simulink model "kopter_se_zavazim_LQR"  (R2024b)
settings: Solver=ode4  StartTime=0.0  StopTime=16  FixedStep=Ts  RelTol=1e-3
values from neighbouring files (symbols this model uses):
  Ac = double(Ac)    [odvozeni_stavova_regulace_a_LQR.m]
  b_moment = 3.6e-7    (= 3.6e-07)    [parametry_kopter_se_zavazim.m]
  Bc = double(Bc)    [odvozeni_stavova_regulace_a_LQR.m]
  Cc = eye(8, 16)    [odvozeni_stavova_regulace_a_LQR.m]
  d = 1    [parametry_kopter_se_zavazim.m]
  Dc = 0    [odvozeni_stavova_regulace_a_LQR.m]
  init_int_dref_lqr = -Ki_lqr\((Uinit-Us)+Kp_lqr*(Xinit_ss-Xs))    [odvozeni_stavova_regulace_a_LQR.m]
  init_int_ref_lqr = -Ki_lqr\(Kp_lqr*xss+uss)    [odvozeni_stavova_regulace_a_LQR.m]
  Ip = m*d^2    (= 1)    [parametry_kopter_se_zavazim.m]
  Ixx = 0.0222    [parametry_kopter_se_zavazim.m]
  Iyy = 0.0222    [parametry_kopter_se_zavazim.m]
  Izz = 0.0429    [parametry_kopter_se_zavazim.m]
  k_thrust = 9.3e-6    (= 9.3e-06)    [parametry_kopter_se_zavazim.m]
  Ki_lqr = K_ex_lqr(:, 17:20)    [odvozeni_stavova_regulace_a_LQR.m]
  Kp_lqr = K_ex_lqr(:, 1:16)    [odvozeni_stavova_regulace_a_LQR.m]
  l = 0.2051    [parametry_kopter_se_zavazim.m]
  M = 2    [parametry_kopter_se_zavazim.m]
  m = 1    [parametry_kopter_se_zavazim.m]
  R_kalman = diag([repmat(1e-2, 1, 3), repmat(7e-4, 1, 3), repmat(3e-4, 1, 2)])    [odvozeni_stavova_regulace_a_LQR.m]
  Ts = 0.01    [odvozeni_stavova_regulace_a_LQR.m]
  Us = [(M+m)*g; 0; 0; 0]    [parametry_kopter_se_zavazim.m]
  Xinit_ss = [Xinit_matrix; [0 0 0 0 0 0 0 0]']    [parametry_kopter_se_zavazim.m]
  Xs = [0;0;0; 0;0;0; 0;0; 0;0;0; 0;0;0; 0;0]    [parametry_kopter_se_zavazim.m]
undefined symbols (not defined in the file or in its folder): Continuous, L, Time
libraries: simulink_extras x11, ctrlSharedLib x2, simulink x2
(part 1 of 3)
settings Model: Creator=Admin  LastModifiedBy=Admin

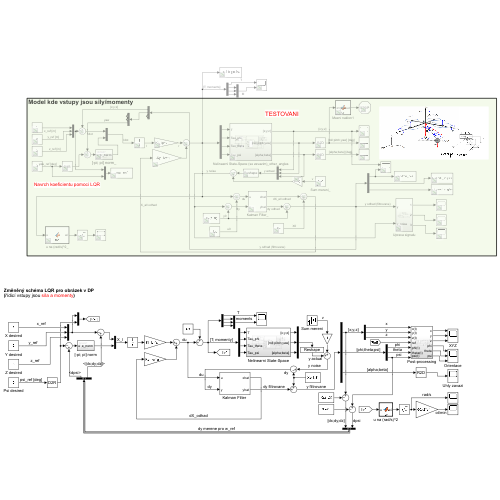
[thumbnail: Simulink's stored preview of the top-level diagram]
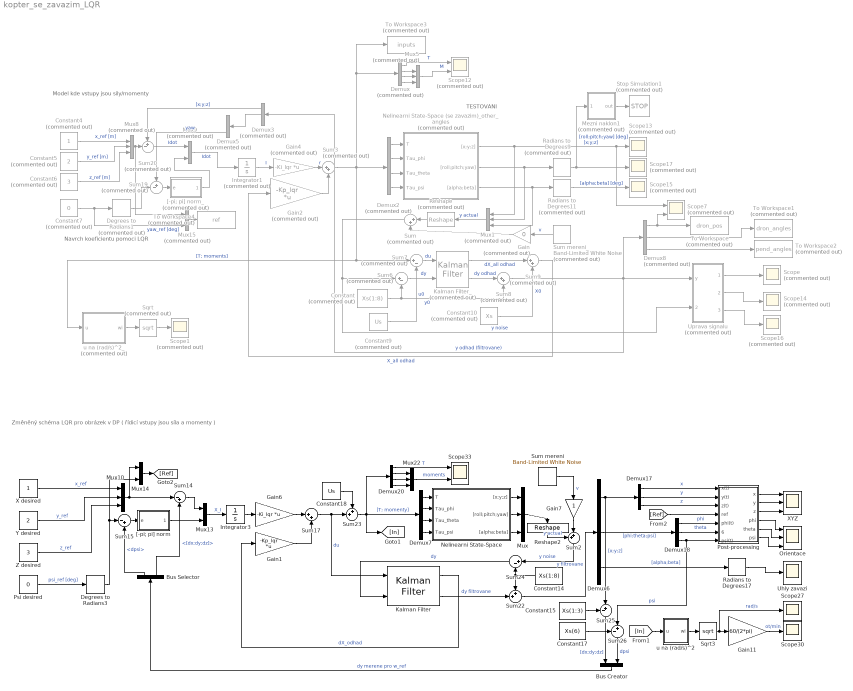
== system kopter_se_zavazim_LQR ==
  note: TESTOVANI
  note: Navrch koeficientu pomoci LQR
  note: Model kde vstupy jsou sily/momenty
  note: Změněný schéma LQR pro obrázek v DP
      | ( řídicí vstupy jsou síla a momenty )
  Bus Creator : BusCreator  Inputs=2
  Bus Selector : BusSelector  OutputSignals=dpsi,[dx;dy;dz]
  Constant : Constant  Commented=on  Value=Xs(1:8)
  Constant10 : Constant  Commented=on  Value=Xs
  Constant14 : Constant  Value=Xs(1:8)
  Constant15 : Constant  Value=Xs(1:3)
  Constant17 : Constant  Value=Xs(6)
  Constant18 : Constant  Value=Us
  Constant4 : Constant  Commented=on
  Constant5 : Constant  Commented=on  Value=2
  Constant6 : Constant  Commented=on  Value=3
  Constant7 : Constant  Commented=on  Value=0
  Constant9 : Constant  Commented=on  Value=Us
  Degrees to Radians1 : simulink_extras/Transformations/Degrees to Radians  Commented=on
  Degrees to Radians3 : simulink_extras/Transformations/Degrees to Radians
  Demux : Demux  Commented=on
  Demux17 : Demux  Outputs=3
  Demux18 : Demux  Outputs=3
  Demux2 : Demux  Commented=on
  Demux20 : Demux
  Demux3 : Demux  Commented=on  Outputs=3
  Demux5 : Demux  Commented=on  Outputs=3
  Demux6 : Demux  Outputs=3
  Demux7 : Demux
  Demux8 : Demux  Commented=on  Outputs=3
  Gain : Gain  Commented=on  Gain=0
  Gain1 : Gain  Gain=-Kp_lqr  Multiplication=Matrix(K*u)
  Gain11 : Gain  Gain=60/(2*pi)
  Gain2 : Gain  Commented=on  Gain=-Kp_lqr  Multiplication=Matrix(K*u)
  Gain4 : Gain  Commented=on  Gain=-Ki_lqr  Multiplication=Matrix(K*u)
  Gain6 : Gain  Gain=-Ki_lqr  Multiplication=Matrix(K*u)
  Gain7 : Gain
  Integrator1 : Integrator  Commented=on  InitialCondition=init_int_ref_lqr
  Integrator3 : Integrator  InitialCondition=init_int_dref_lqr
  "Kalman Filter " : ctrlSharedLib/Kalman Filter  TimeDomain=Continuous-Time  UseCurrentEstimator=on  ModelSource=Individual A, B, C, D matrices  ModelSourceVariable=ss(0.95,1,1,0,1)  A=Ac  B=Bc  C=Cc  D=Dc  NumberOfStates=1  NumberOfInputs=1  NumberOfOutputs=1  InitialEstimateSource=Dialog  X0=Xinit_ss-Xs  P0=10  UseK=off  UseGH=off  NumberOfProcessNoiseInputs=1  G=1  TimeInvariantG=on  H=0  TimeInvariantH=on  Q=Q_kalman  TimeInvariantQ=on  R=R_kalman  TimeInvariantR=on  N=0  TimeInvariantN=on  AddInputPort=on  AddEnablePort=off  OutputEstimatedY=on  OutputP=off  Ts=-1
  Kalman Filter_ : ctrlSharedLib/Kalman Filter  Commented=on  TimeDomain=Continuous-Time  UseCurrentEstimator=on  ModelSource=Individual A, B, C, D matrices  ModelSourceVariable=ss(0.95,1,1,0,1)  A=Ac  B=Bc  C=Cc  D=Dc  NumberOfStates=1  NumberOfInputs=1  NumberOfOutputs=1  InitialEstimateSource=Dialog  X0=Xinit_ss-Xs  P0=10  UseK=off  UseGH=off  NumberOfProcessNoiseInputs=1  G=1  TimeInvariantG=on  H=0  TimeInvariantH=on  Q=Q_kalman  TimeInvariantQ=on  R=R_kalman  TimeInvariantR=on  N=0  TimeInvariantN=on  AddInputPort=on  AddEnablePort=off  OutputEstimatedY=on  OutputP=off  Ts=-1
  Mezni naklon1 : MATLAB Function  Commented=on  TreatAsAtomicUnit=on
  Mux : Mux  Inputs=3
  Mux1 : Mux  Commented=on  Inputs=3
  Mux10 : Mux  Inputs=3
  Mux13 : Mux  Inputs=2
  Mux14 : Mux  Inputs=2
  Mux15 : Mux  Commented=on  Inputs=2
  Mux22 : Mux  Inputs=3
  Mux5 : Mux  Commented=on  Inputs=3
  Mux8 : Mux  Commented=on  Inputs=3
  Mux9 : Mux  Commented=on  Inputs=2
  Nelinearni State-Space : Subsystem
  Nelinearni State-Space (se zavazim)_other_angles : Subsystem  Commented=on
  Orientace : Scope  NumInputPorts=3
  Post-processing : Subsystem
  Psi desired : Constant  Value=0
  Radians to Degrees11 : simulink_extras/Transformations/Radians to Degrees  Commented=on
  Radians to Degrees17 : simulink_extras/Transformations/Radians to Degrees
  Radians to Degrees9 : simulink_extras/Transformations/Radians to Degrees  Commented=on
  Reshape : Reshape  Commented=on  OutputDimensionality=Customize  OutputDimensions=[8,1]
  Reshape2 : Reshape  OutputDimensionality=Customize  OutputDimensions=[8,1]
  Scope{,1,13..17} (7 alike) : Scope  Commented=on
  Scope12 : Scope  Commented=on  NumInputPorts=2
  Scope27 : Scope
  Scope30 : Scope
  Scope33 : Scope  NumInputPorts=2
  Scope7 : Scope  Commented=on  NumInputPorts=2
  Sqrt : Sqrt  Commented=on
  Sqrt3 : Sqrt
  Stop Simulation1 : Stop  Commented=on
  Sum{,3,8..9} (4 alike) : Sum  Commented=on  Inputs=|++
  Sum mereni : simulink/Sources/Band-Limited White Noise  Cov=diag(R_kalman)*Ts  Ts=Ts  seed=[23341]
  Sum mereni_ : simulink/Sources/Band-Limited White Noise  Commented=on  Cov=diag(R_kalman)*Ts  Ts=Ts  seed=[23341]
  Sum14 : Sum  Inputs=|-+
  Sum15 : Sum  Inputs=|-+
  Sum17 : Sum  Inputs=|++
  Sum19 : Sum  Commented=on  Inputs=+-|
  Sum2 : Sum  Inputs=++|
  Sum20 : Sum  Commented=on  Inputs=+-|
  Sum22 : Sum  Inputs=++|
  Sum23 : Sum  Inputs=++|
  Sum24 : Sum  Inputs=|+-
  Sum25 : Sum  Inputs=-+|
  Sum26 : Sum  Inputs=-+|
  Sum6 : Sum  Commented=on  Inputs=|+-
  Sum7 : Sum  Commented=on  Inputs=|+-
  To Workspace : ToWorkspace  Commented=on  VariableName=dron_pos  SaveFormat=Timeseries  SampleTime=-1
  To Workspace1 : ToWorkspace  Commented=on  VariableName=dron_angles  SaveFormat=Timeseries  SampleTime=-1
  To Workspace2 : ToWorkspace  Commented=on  VariableName=pend_angles  SaveFormat=Timeseries  SampleTime=-1
  To Workspace3 : ToWorkspace  Commented=on  VariableName=inputs  SaveFormat=Timeseries  SampleTime=-1
  To Workspace4 : ToWorkspace  Commented=on  VariableName=ref  SaveFormat=Timeseries  SampleTime=-1
  Uhly zavazi : Scope
  Uprava signalu : Subsystem  Commented=on
  X desired : Constant
  XYZ : Scope  NumInputPorts=3
  Y desired : Constant  Value=2
  Z desired : Constant  Value=3
  "[-pi; pi] norm" : Subsystem
  "[-pi; pi] norm_" : Subsystem  Commented=on
  u na (rad/s)^2 : MATLAB Function  TreatAsAtomicUnit=on
  u na (rad/s)^2_ : MATLAB Function  Commented=on  TreatAsAtomicUnit=on
  wires:
  Nelinearni State-Space (se zavazim)_other_angles/3("[alpha;beta]") -> Radians to Degrees11/1, Mux1/3
  Radians to Degrees9/1 -> Scope17/1, Mezni naklon1/1(angles)  "[roll;pitch;yaw] [deg]"
  Radians to Degrees11/1 -> Scope15/1  "[alpha;beta] [deg]"
  Demux2/3 -> Nelinearni State-Space (se zavazim)_other_angles/3(Tau_theta)
  Demux2/2 -> Nelinearni State-Space (se zavazim)_other_angles/2(Tau_phi)
  Constant5/1 -> Mux8/2  "y_ref [m]"
  Constant6/1 -> Mux8/3  "z_ref [m]"
  Gain2/1 -> Sum3/2
  Demux2/4 -> Nelinearni State-Space (se zavazim)_other_angles/4(Tau_psi)
  Gain4/1 -> Sum3/1  "r"
  Demux2/1 -> Nelinearni State-Space (se zavazim)_other_angles/1(T)
  Integrator1/1 -> Gain4/1  "I"
  Degrees to Radians1/1 -> Sum19/2
  Constant4/1 -> Mux8/1  "x_ref [m]"
  Nelinearni State-Space (se zavazim)_other_angles/1("[x;y;z]") -> Scope7/1, Scope13/1, Mux1/1  "[x;y;z]"
  Nelinearni State-Space (se zavazim)_other_angles/2("[roll;pitch;yaw]") -> Radians to Degrees9/1, Mux1/2
  Mezni naklon1/1(out) -> Stop Simulation1/1
  u na (rad/s)^2_/1(wi) -> Sqrt/1
  Mux1/1 -> Reshape/1  "y actual"
  Sum mereni_/1 -> Gain/1  "v"
  Kalman Filter_/1 -> Sum9/1  "dX_all odhad"
  Kalman Filter_/2 -> Sum8/1  "dy odhad"
  Reshape/1 -> Sum/1
  Sum6/1 -> Kalman Filter_/2  "dy"
  Constant/1 -> Sum8/2, Sum6/2  "y0"
  Sum7/1 -> Kalman Filter_/1  "du"
  Constant9/1 -> Sum7/2  "u0"
  Sum8/1 -> Demux3/1, Demux8/1, Uprava signalu/1(y)  "y odhad (filtrovane)"
  Constant10/1 -> Sum9/2  "X0"
  Sum9/1 -> Gain2/1  "X_all odhad"
  Radians to Degrees17/1 -> Uhly zavazi/1
  Post-processing/6(psi) -> Orientace/3
  Post-processing/5(theta) -> Orientace/2
  Demux7/2 -> Nelinearni State-Space/2(Tau_phi)
  [Ref] -> Post-processing/4(ref)
  Demux18/2 -> Post-processing/6(theta(t))  "theta"
  Y desired/1 -> Mux10/2  "y_ref"
  Demux17/2 -> Post-processing/2(y(t))  "y"
  Demux18/3 -> Sum26/2, Post-processing/7(psi(t))  "psi"
  Bus Creator/1 -> Bus Selector/1  "dy merene pro w_ref"
  Post-processing/4(phi) -> Orientace/1
  Mux22/1 -> Scope33/2  "moments"
  Sum23/1 -> [In], Demux7/1, Demux20/1  "[T; momenty]"
  Mux13/1 -> Integrator3/1  "X_I"
  Demux18/1 -> Post-processing/5(phi(t))  "phi"
  Demux17/3 -> Post-processing/3(z(t))  "z"
  Gain11/1 -> Scope30/1  "ot/min"
  X desired/1 -> Mux10/1  "x_ref"
  [In] -> u na (rad/s)^2/1(u)
  Post-processing/1(x) -> XYZ/1
  Gain6/1 -> Sum17/1
  "[-pi; pi] norm"/1(e_norm) -> Mux13/2
  Demux20/4 -> Mux22/3
  Degrees to Radians3/1 -> Mux14/2, Sum15/1
  Sum14/1 -> Mux13/1
  Demux6/3 -> Radians to Degrees17/1  "[alpha;beta]"
  Demux20/1 -> Scope33/1  "T"
  Demux20/3 -> Mux22/2
  Z desired/1 -> Mux10/3  "z_ref"
  Demux17/1 -> Post-processing/1(x(t))  "x"
  Post-processing/2(y) -> XYZ/2
  Sum15/1 -> "[-pi; pi] norm"/1(e)
  Mux10/1 -> Mux14/1, Sum14/1
  u na (rad/s)^2/1(wi) -> Sqrt3/1
  Post-processing/3(z) -> XYZ/3
  Demux7/4 -> Nelinearni State-Space/4(Tau_psi)
  Integrator3/1 -> Gain6/1
  Demux6/1 -> Sum25/2, Demux17/1  "[x;y;z]"
  Gain1/1 -> Sum17/2
  Mux14/1 -> [Ref]
  Sqrt3/1 -> Scope27/1, Gain11/1  "rad/s"
  Psi desired/1 -> Degrees to Radians3/1  "psi_ref [deg]"
  Demux7/3 -> Nelinearni State-Space/3(Tau_theta)
  Demux20/2 -> Mux22/1
  Demux7/1 -> Nelinearni State-Space/1(T)
  Demux6/2 -> Demux18/1  "[phi;theta;psi]"
  Sqrt/1 -> Scope1/1
  Sum3/1 -> Demux2/1, Demux/1, To Workspace3/1, Sum7/1, u na (rad/s)^2_/1(u)  "[T; moments]"
  Demux/2 -> Mux5/1
  Demux/3 -> Mux5/2
  Demux/4 -> Mux5/3
  Mux5/1 -> Scope12/2  "M"
  Demux/1 -> Scope12/1  "T"
  Constant7/1 -> Mux15/2, Degrees to Radians1/1  "yaw_ref [deg]"
  Mux9/1 -> Integrator1/1  "Idot"
  Sum20/1 -> Mux9/1  "Idot"
  Sum19/1 -> "[-pi; pi] norm_"/1(e)
  "[-pi; pi] norm_"/1(e_norm) -> Mux9/2
  Uprava signalu/1(Output) -> Scope/1
  Uprava signalu/3(Output2) -> Scope16/1
  Sum/1 -> Sum6/1, Uprava signalu/2(y_noise)  "y noise"
  Demux3/2 -> Demux5/1
  Demux3/1 -> Sum20/1  "[x;y;z]"
  Demux5/3 -> Sum19/1  "yaw"
  Uprava signalu/2(Output1) -> Scope14/1
  Reshape2/1 -> Sum2/1  "y actual"
  Sum mereni/1 -> Gain7/1  "v"
  Sum2/1 -> Sum24/1  "y noise"
  "Kalman Filter "/1 -> Gain1/1  "dX_odhad"
  Sum17/1 -> "Kalman Filter "/1, Sum23/2  "du"
  Nelinearni State-Space/1("[x;y;z]") -> Mux/1
  Nelinearni State-Space/2("[roll;pitch;yaw]") -> Mux/2
  Nelinearni State-Space/3("[alpha;beta]") -> Mux/3
  Mux/1 -> Reshape2/1
  "Kalman Filter "/2 -> Sum22/2  "dy filtrovane"
  Sum22/1 -> Demux6/1  "y filtrovane"
  Mux8/1 -> Mux15/1, Sum20/2
  Mux15/1 -> To Workspace4/1
  Demux8/2 -> To Workspace1/1
  Demux8/1 -> To Workspace/1, Scope7/2
  Demux8/3 -> To Workspace2/1
  Gain/1 -> Sum/2
  Constant18/1 -> Sum23/1
  Sum24/1 -> "Kalman Filter "/2  "dy"
  Constant14/1 -> Sum22/1, Sum24/2
  Constant15/1 -> Sum25/1
  Constant17/1 -> Sum26/1
  Sum26/1 -> Bus Creator/2  "dpsi"
  Sum25/1 -> Bus Creator/1  "[dx;dy;dz]"
  Bus Selector/1 -> Sum15/2  "<dpsi>"
  Bus Selector/2 -> Sum14/2  "<[dx;dy;dz]>"
  Gain7/1 -> Sum2/2

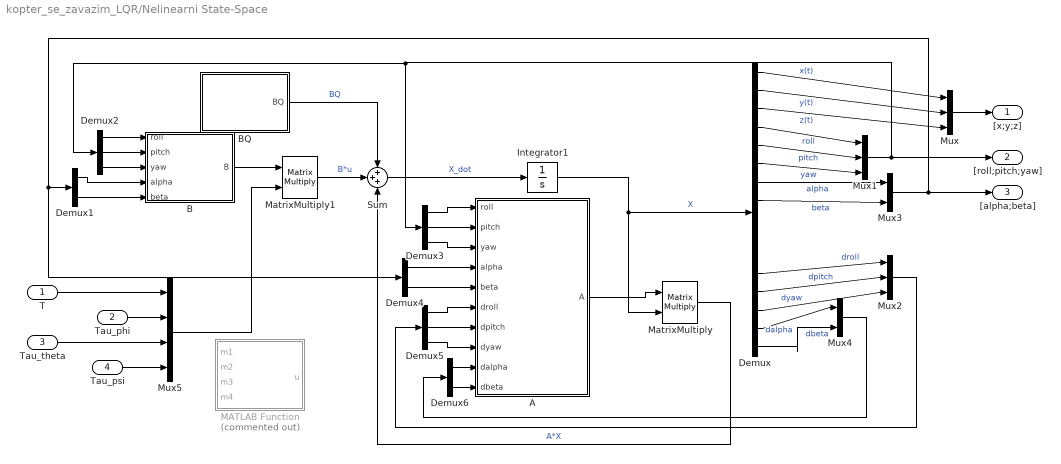
== system kopter_se_zavazim_LQR/Nelinearni State-Space ==
  T : Inport
  Tau_phi : Inport  Port=2
  Tau_theta : Inport  Port=3
  Tau_psi : Inport  Port=4
  A : MATLAB Function  TreatAsAtomicUnit=on
  B : MATLAB Function  TreatAsAtomicUnit=on
  BQ : MATLAB Function  TreatAsAtomicUnit=on
  Demux : Demux  Outputs=16
  Demux1 : Demux  Outputs=2
  Demux2 : Demux  Outputs=3
  Demux3 : Demux  Outputs=3
  Demux4 : Demux  Outputs=2
  Demux5 : Demux  Outputs=3
  Demux6 : Demux  Outputs=2
  Integrator1 : Integrator  InitialCondition=Xinit_ss
  MATLAB Function : MATLAB Function  Commented=on  TreatAsAtomicUnit=on
  MatrixMultiply : Product  Multiplication=Matrix(*)
  MatrixMultiply1 : Product  Multiplication=Matrix(*)
  Mux : Mux  Inputs=3
  Mux1 : Mux  Inputs=3
  Mux2 : Mux  Inputs=3
  Mux3 : Mux  Inputs=2
  Mux4 : Mux  Inputs=2
  Mux5 : Mux
  Sum : Sum  Inputs=+++
  "[x;y;z]" : Outport
  "[roll;pitch;yaw]" : Outport  Port=2
  "[alpha;beta]" : Outport  Port=3
  wires:
  A/1(A) -> MatrixMultiply/1
  Integrator1/1 -> MatrixMultiply/2, Demux/1  "X"
  Demux/1 -> Mux/1  "x(t)"
  Demux/2 -> Mux/2  "y(t)"
  Demux/3 -> Mux/3  "z(t)"
  Mux/1 -> "[x;y;z]"/1
  Demux/4 -> Mux1/1  "roll"
  Demux/5 -> Mux1/2  "pitch"
  Demux/6 -> Mux1/3  "yaw"
  Mux1/1 -> Demux2/1, Demux3/1, "[roll;pitch;yaw]"/1
  Demux/12 -> Mux2/1  "droll"
  Demux/13 -> Mux2/2  "dpitch"
  Demux/14 -> Mux2/3  "dyaw"
  Demux2/1 -> B/1(roll)
  Demux2/2 -> B/2(pitch)
  Demux2/3 -> B/3(yaw)
  Demux3/2 -> A/2(pitch)
  Demux3/1 -> A/1(roll)
  Demux3/3 -> A/3(yaw)
  Demux5/2 -> A/7(dpitch)
  Demux5/1 -> A/6(droll)
  Demux5/3 -> A/8(dyaw)
  Sum/1 -> Integrator1/1  "X_dot"
  BQ/1(BQ) -> Sum/1  "BQ"
  MatrixMultiply1/1 -> Sum/2  "B*u"
  B/1(B) -> MatrixMultiply1/1
  MatrixMultiply/1 -> Sum/3  "A*X"
  Mux2/1 -> Demux5/1
  Demux/7 -> Mux3/1  "alpha"
  Demux/8 -> Mux3/2  "beta"
  Mux3/1 -> Demux4/1, Demux1/1, "[alpha;beta]"/1
  Demux1/2 -> B/5(beta)
  Demux1/1 -> B/4(alpha)
  Demux4/2 -> A/5(beta)
  Demux4/1 -> A/4(alpha)
  Demux/15 -> Mux4/1  "dalpha"
  Demux/16 -> Mux4/2  "dbeta"
  Demux6/1 -> A/9(dalpha)
  Demux6/2 -> A/10(dbeta)
  Mux4/1 -> Demux6/1
  Tau_theta/1 -> Mux5/3
  Tau_psi/1 -> Mux5/4
  Tau_phi/1 -> Mux5/2
  Mux5/1 -> MatrixMultiply1/2
  T/1 -> Mux5/1

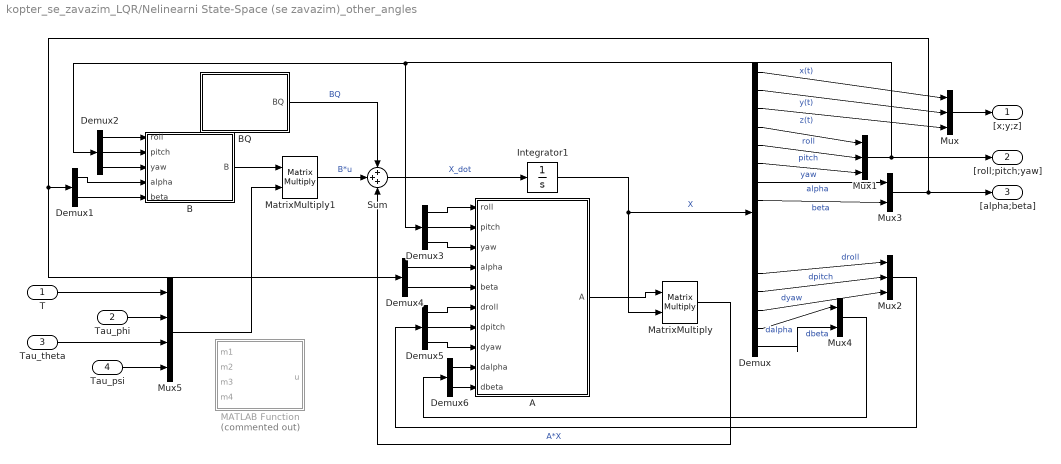
== system kopter_se_zavazim_LQR/Nelinearni State-Space (se zavazim)_other_angles ==
  T : Inport
  Tau_phi : Inport  Port=2
  Tau_theta : Inport  Port=3
  Tau_psi : Inport  Port=4
  A : MATLAB Function  TreatAsAtomicUnit=on
  B : MATLAB Function  TreatAsAtomicUnit=on
  BQ : MATLAB Function  TreatAsAtomicUnit=on
  Demux : Demux  Outputs=16
  Demux1 : Demux  Outputs=2
  Demux2 : Demux  Outputs=3
  Demux3 : Demux  Outputs=3
  Demux4 : Demux  Outputs=2
  Demux5 : Demux  Outputs=3
  Demux6 : Demux  Outputs=2
  Integrator1 : Integrator  InitialCondition=Xinit_ss
  MATLAB Function : MATLAB Function  Commented=on  TreatAsAtomicUnit=on
  MatrixMultiply : Product  Multiplication=Matrix(*)
  MatrixMultiply1 : Product  Multiplication=Matrix(*)
  Mux : Mux  Inputs=3
  Mux1 : Mux  Inputs=3
  Mux2 : Mux  Inputs=3
  Mux3 : Mux  Inputs=2
  Mux4 : Mux  Inputs=2
  Mux5 : Mux
  Sum : Sum  Inputs=+++
  "[x;y;z]" : Outport
  "[roll;pitch;yaw]" : Outport  Port=2
  "[alpha;beta]" : Outport  Port=3
  wires:
  A/1(A) -> MatrixMultiply/1
  Integrator1/1 -> MatrixMultiply/2, Demux/1  "X"
  Demux/1 -> Mux/1  "x(t)"
  Demux/2 -> Mux/2  "y(t)"
  Demux/3 -> Mux/3  "z(t)"
  Mux/1 -> "[x;y;z]"/1
  Demux/4 -> Mux1/1  "roll"
  Demux/5 -> Mux1/2  "pitch"
  Demux/6 -> Mux1/3  "yaw"
  Mux1/1 -> Demux2/1, Demux3/1, "[roll;pitch;yaw]"/1
  Demux/12 -> Mux2/1  "droll"
  Demux/13 -> Mux2/2  "dpitch"
  Demux/14 -> Mux2/3  "dyaw"
  Demux2/1 -> B/1(roll)
  Demux2/2 -> B/2(pitch)
  Demux2/3 -> B/3(yaw)
  Demux3/2 -> A/2(pitch)
  Demux3/1 -> A/1(roll)
  Demux3/3 -> A/3(yaw)
  Demux5/2 -> A/7(dpitch)
  Demux5/1 -> A/6(droll)
  Demux5/3 -> A/8(dyaw)
  Sum/1 -> Integrator1/1  "X_dot"
  BQ/1(BQ) -> Sum/1  "BQ"
  MatrixMultiply1/1 -> Sum/2  "B*u"
  B/1(B) -> MatrixMultiply1/1
  MatrixMultiply/1 -> Sum/3  "A*X"
  Mux2/1 -> Demux5/1
  Demux/7 -> Mux3/1  "alpha"
  Demux/8 -> Mux3/2  "beta"
  Mux3/1 -> Demux4/1, Demux1/1, "[alpha;beta]"/1
  Demux1/2 -> B/5(beta)
  Demux1/1 -> B/4(alpha)
  Demux4/2 -> A/5(beta)
  Demux4/1 -> A/4(alpha)
  Demux/15 -> Mux4/1  "dalpha"
  Demux/16 -> Mux4/2  "dbeta"
  Demux6/1 -> A/9(dalpha)
  Demux6/2 -> A/10(dbeta)
  Mux4/1 -> Demux6/1
  Tau_theta/1 -> Mux5/3
  Tau_psi/1 -> Mux5/4
  Tau_phi/1 -> Mux5/2
  Mux5/1 -> MatrixMultiply1/2
  T/1 -> Mux5/1

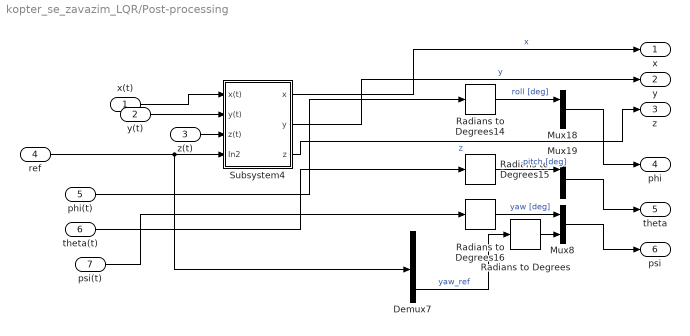
== system kopter_se_zavazim_LQR/Post-processing ==
  x(t) : Inport
  y(t) : Inport  Port=2
  z(t) : Inport  Port=3
  ref : Inport  Port=4
  phi(t) : Inport  Port=5
  theta(t) : Inport  Port=6
  psi(t) : Inport  Port=7
  Demux7 : Demux
  Mux18 : Mux  Inputs=2
  Mux19 : Mux  Inputs=2
  Mux8 : Mux  Inputs=2
  Radians to Degrees{,14..16} (4 alike) : simulink_extras/Transformations/Radians to Degrees
  Subsystem4 : Subsystem
  x : Outport
  y : Outport  Port=2
  z : Outport  Port=3
  phi : Outport  Port=4
  theta : Outport  Port=5
  psi : Outport  Port=6
  wires:
  Radians to Degrees16/1 -> Mux8/1  "yaw [deg]"
  ref/1 -> Subsystem4/4(In2), Demux7/1
  Demux7/4 -> Radians to Degrees/1  "yaw_ref"
  theta(t)/1 -> Radians to Degrees15/1
  Mux18/1 -> phi/1
  Subsystem4/3(z) -> z/1  "z"
  Radians to Degrees14/1 -> Mux18/1  "roll [deg]"
  Radians to Degrees15/1 -> Mux19/1  "pitch [deg]"
  Subsystem4/2(y) -> y/1  "y"
  x(t)/1 -> Subsystem4/1(x(t))
  y(t)/1 -> Subsystem4/2(y(t))
  psi(t)/1 -> Radians to Degrees16/1
  phi(t)/1 -> Radians to Degrees14/1
  Subsystem4/1(x) -> x/1  "x"
  Mux8/1 -> psi/1
  z(t)/1 -> Subsystem4/3(z(t))
  Mux19/1 -> theta/1
  Radians to Degrees/1 -> Mux8/2

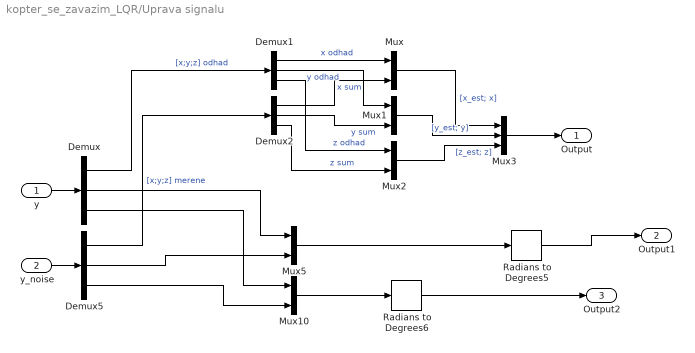
== system kopter_se_zavazim_LQR/Uprava signalu ==
  y : Inport
  y_noise : Inport  Port=2
  Demux{,1..2,5} (4 alike) : Demux  Outputs=3
  Mux{,1..2,5,10} (5 alike) : Mux  Inputs=2
  Mux3 : Mux  Inputs=3
  Radians to Degrees5 : simulink_extras/Transformations/Radians to Degrees
  Radians to Degrees6 : simulink_extras/Transformations/Radians to Degrees
  Output : Outport
  Output1 : Outport  Port=2
  Output2 : Outport  Port=3
  wires:
  Demux5/3 -> Mux10/2
  Demux/3 -> Mux10/1
  Mux5/1 -> Radians to Degrees5/1
  Demux/2 -> Mux5/1
  Demux5/2 -> Mux5/2
  Demux5/1 -> Demux2/1  "[x;y;z] merene"
  Demux/1 -> Demux1/1  "[x;y;z] odhad"
  Mux10/1 -> Radians to Degrees6/1
  y/1 -> Demux/1
  Radians to Degrees5/1 -> Output1/1
  y_noise/1 -> Demux5/1
  Demux1/1 -> Mux/1  "x odhad"
  Demux2/1 -> Mux/2  "x sum"
  Demux1/2 -> Mux1/1  "y odhad"
  Demux2/2 -> Mux1/2  "y sum"
  Mux/1 -> Mux3/1  "[x_est; x]"
  Mux1/1 -> Mux3/2  "[y_est; y]"
  Mux2/1 -> Mux3/3  "[z_est; z]"
  Demux1/3 -> Mux2/1  "z odhad"
  Demux2/3 -> Mux2/2  "z sum"
  Mux3/1 -> Output/1
  Radians to Degrees6/1 -> Output2/1

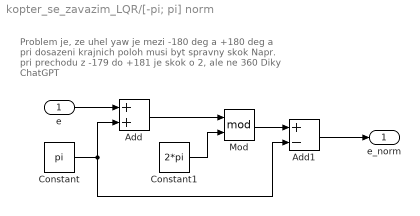
== system kopter_se_zavazim_LQR/[-pi; pi] norm ==
  note: Problem je, ze uhel yaw je mezi -180 deg a +180 deg
      | a pri dosazeni krajnich poloh musi byt spravny skok
      | Napr. pri prechodu z -179 do +181 je skok o 2, ale ne 360
      | Diky ChatGPT
  e : Inport
  Add : Sum
  Add1 : Sum  Inputs=+-
  Constant : Constant  Value=pi
  Constant1 : Constant  Value=2*pi
  Mod : Math  Operator=mod
  e_norm : Outport
  wires:
  e/1 -> Add/1
  Add/1 -> Mod/1
  Constant/1 -> Add1/2, Add/2
  Constant1/1 -> Mod/2
  Mod/1 -> Add1/1
  Add1/1 -> e_norm/1

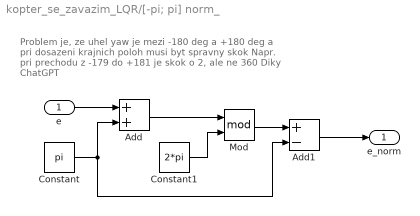
== system kopter_se_zavazim_LQR/[-pi; pi] norm_ ==
  note: Problem je, ze uhel yaw je mezi -180 deg a +180 deg
      | a pri dosazeni krajnich poloh musi byt spravny skok
      | Napr. pri prechodu z -179 do +181 je skok o 2, ale ne 360
      | Diky ChatGPT
  e : Inport
  Add : Sum
  Add1 : Sum  Inputs=+-
  Constant : Constant  Value=pi
  Constant1 : Constant  Value=2*pi
  Mod : Math  Operator=mod
  e_norm : Outport
  wires:
  e/1 -> Add/1
  Add/1 -> Mod/1
  Constant/1 -> Add1/2, Add/2
  Constant1/1 -> Mod/2
  Mod/1 -> Add1/1
  Add1/1 -> e_norm/1

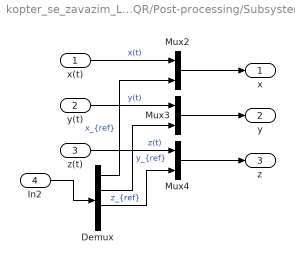
== system kopter_se_zavazim_LQR/Post-processing/Subsystem4 ==
  x(t) : Inport
  y(t) : Inport  Port=2
  z(t) : Inport  Port=3
  In2 : Inport  Port=4
  Demux : Demux
  Mux2 : Mux  Inputs=2
  Mux3 : Mux  Inputs=2
  Mux4 : Mux  Inputs=2
  x : Outport
  y : Outport  Port=2
  z : Outport  Port=3
  wires:
  Demux/2 -> Mux3/2  "y_{ref}"
  Mux4/1 -> z/1
  y(t)/1 -> Mux3/1  "y(t)"
  Mux3/1 -> y/1
  Demux/1 -> Mux2/2  "x_{ref}"
  Demux/3 -> Mux4/2  "z_{ref}"
  Mux2/1 -> x/1
  In2/1 -> Demux/1
  x(t)/1 -> Mux2/1  "x(t)"
  z(t)/1 -> Mux4/1  "z(t)"

== matlab function kopter_se_zavazim_LQR/u na (rad//s)^2 ==
  data: u input; wi output; b_moment parameter; k_thrust parameter; l parameter
function wi = fcn(u, b_moment, k_thrust, l)

T = u(1);
Tau_phi = u(2);
Tau_theta = u(3);
Tau_psi = u(4);

w1 = ( (Tau_phi*b_moment - Tau_theta*b_moment + l*T*b_moment + l*Tau_psi*k_thrust)/(4*l*b_moment*k_thrust));
w2 = ( (-Tau_theta*b_moment - Tau_phi*b_moment + l*T*b_moment - l*Tau_psi*k_thrust)/(4*l*b_moment*k_thrust));
w3 = ( (Tau_theta*b_moment - Tau_phi*b_moment + l*T*b_moment + l*Tau_psi*k_thrust)/(4*l*b_moment*k_thrust));
w4 = ( (Tau_phi*b_moment + Tau_theta*b_moment + l*T*b_moment - l*Tau_psi*k_thrust)/(4*l*b_moment*k_thrust));

wi = [w1;w2;w3;w4];

== matlab function kopter_se_zavazim_LQR/Nelinearni State-Space (se zavazim)_other_angles/A ==
  data: roll input; A output; pitch input; yaw input; alpha input; beta input; droll input; dpitch input; dyaw input; dalpha input; dbeta input; Ixx parameter; Iyy parameter; Izz parameter; M parameter; Ip parameter; d parameter; m parameter
function A = fcn(roll, pitch, yaw, alpha, beta, droll, dpitch, dyaw, dalpha, dbeta, Ixx, Iyy, Izz, M, Ip, d, m)
% Matice dynamiky A

phi_t = roll;
theta_t = pitch;
psi_t = yaw;

alpha_t = alpha;
beta_t = beta;

phi_dot_t = droll;
theta_dot_t = dpitch;
psi_dot_t = dyaw;

alpha_dot_t = dalpha;
beta_dot_t = dbeta;

A = [ 
0, 0, 0, 0, 0, 0, 0, 0, 1, 0, 0,                                                                                                                                                                                                                                                                                                                                                                                                                                                                                                           0,                                                                                                                                                                                                                                                                                                                                                                                                                                                                                                                                                                                                                                                                                                                              0,                                                                                                                                                                                            0,                                                          0,                                                  0;
0, 0, 0, 0, 0, 0, 0, 0, 0, 1, 0,                                                                                                                                                                                                                                                                                                                                                                                                                                                                                                           0,                                                                                                                                                                                                                                                                                                                                                                                                                                                                                                                                                                                                                                                                                                                              0,                                                                                                                                                                                            0,                                                          0,                                                  0;
0, 0, 0, 0, 0, 0, 0, 0, 0, 0, 1,                                                                                                                                                                                                                                                                                                                                                                                                                                                                                                           0,                                                                                                                                                                                                                                                                                                                                                                                                                                                                                                                                                                                                                                                                                                                              0,                                                                                                                                                                                            0,                                                          0,                                                  0;
0, 0, 0, 0, 0, 0, 0, 0, 0, 0, 0,                                                                                                                                                                                                                                                                                                                                                                                                                                                                                                           1,                                                                                                                                                                                                                                                                                                                                                                                                                                                                                                                                                                                                                                                                                                                              0,                                                                                                                                                                                            0,                                                          0,                                                  0;
0, 0, 0, 0, 0, 0, 0, 0, 0, 0, 0,                                                                                                                                                                                                                                                                                                                                                                                                                                                                                                           0,                                                                                                                                                                                                                                                                                                                                                                                                                                                                                                                                                                                                                                                                                                                              1,                                                                                                                                                                                            0,                                                          0,                                                  0;
0, 0, 0, 0, 0, 0, 0, 0, 0, 0, 0,                                                                                                                                                                                                                                                                                                                                                                                                                                                                                                           0,                                                                                                                                                                                                                                                                                                                                                                                                                                                                                                                                                                                                                                                                                                                              0,                                                                                                                                                                                            1,                                                          0,                                                  0;
0, 0, 0, 0, 0, 0, 0, 0, 0, 0, 0,                                                                                                                                                                                                                                                                                                                                                                                                                                                                                                           0,                                                                                                                                                                                                                                                                                                                                                                                                                                                                                                                                                                                                                                                                                                                              0,                                                                                                                                                                                            0,                                                          1,                                                  0;
0, 0, 0, 0, 0, 0, 0, 0, 0, 0, 0,                                                                                                                                                                                                                                                                                                                                                                                                                                                                                                           0,                                                                                                                                                                                                                                                                                                                                                                                                                                                                                                                                                                                                                                                                                                                              0,                                                                                                                                                                                            0,                                                          0,                                                  1;
0, 0, 0, 0, 0, 0, 0, 0, 0, 0, 0,                                                                                                                                                                                                                                                                                                                                                                                                                                                                                                           0,                                                                                                                                                                                                                                                                                                                                                                                                                                                                                                                                                                                                                                                                                                                              0,                                                                                                                                                                                            0,       (alpha_dot_t*d*m*cos(beta_t)^3*sin(alpha_t))/(M + m),  (beta_dot_t*d*m*cos(beta_t)*sin(alpha_t))/(M + m);
0, 0, 0, 0, 0, 0, 0, 0, 0, 0, 0,                                                                                                                                                                                                                                                                                                                                                                                                                                                                                                           0,                                                                                                                                                                                                                                                                                                                                                                                                                                                                                                                                                                                                                                                                                                                              0,                                                                                                                                                                                            0, -(alpha_dot_t*d*m*sin(beta_t)*(sin(beta_t)^2 - 1))/(M + m),               (beta_dot_t*d*m*sin(beta_t))/(M + m);
0, 0, 0, 0, 0, 0, 0, 0, 0, 0, 0,                                                                                                                                                                                                                                                                                                                                                                                                                                                                                                           0,                                                                                                                                                                                                                                                                                                                                                                                                                                                                                                                                                                                                                                                                                                                              0,                                                                                                                                                                                            0,      -(alpha_dot_t*d*m*cos(alpha_t)*cos(beta_t)^3)/(M + m), -(beta_dot_t*d*m*cos(alpha_t)*cos(beta_t))/(M + m);
0, 0, 0, 0, 0, 0, 0, 0, 0, 0, 0,                                       (sin(theta_t)*(Ixx*Izz*theta_dot_t - Izz^2*theta_dot_t + Iyy*Izz*theta_dot_t - Iyy^2*theta_dot_t*cos(phi_t)^2 + Izz^2*theta_dot_t*cos(phi_t)^2 + Ixx*Iyy*theta_dot_t*cos(phi_t)^2 - Ixx*Izz*theta_dot_t*cos(phi_t)^2 - Iyy^2*psi_dot_t*cos(phi_t)*cos(theta_t)*sin(phi_t) + Izz^2*psi_dot_t*cos(phi_t)*cos(theta_t)*sin(phi_t) + Ixx*Iyy*psi_dot_t*cos(phi_t)*cos(theta_t)*sin(phi_t) - Ixx*Izz*psi_dot_t*cos(phi_t)*cos(theta_t)*sin(phi_t)))/(Iyy*Izz*cos(theta_t)), - ((Iyy*Izz + Ixx*Iyy*sin(theta_t)^2 - Iyy*Izz*sin(theta_t)^2 - Ixx*Iyy*sin(phi_t)^2*sin(theta_t)^2 + Ixx*Izz*sin(phi_t)^2*sin(theta_t)^2)*((Izz*theta_dot_t*sin(2*phi_t))/2 - (Iyy*theta_dot_t*sin(2*phi_t))/2 + Ixx*psi_dot_t*cos(theta_t) - Iyy*psi_dot_t*cos(theta_t) + Izz*psi_dot_t*cos(theta_t) + 2*Iyy*psi_dot_t*cos(phi_t)^2*cos(theta_t) - 2*Izz*psi_dot_t*cos(phi_t)^2*cos(theta_t)))/(Ixx*Iyy*Izz*(sin(theta_t)^2 - 1)) - (sin(theta_t)^2*(Iyy - Iyy*sin(phi_t)^2 + Izz*sin(phi_t)^2)*((Iyy*theta_dot_t*sin(2*phi_t))/2 - (Izz*theta_dot_t*sin(2*phi_t))/2 - 2*Ixx*psi_dot_t*cos(theta_t) + 2*Izz*psi_dot_t*cos(phi_t)^2*cos(theta_t) + 2*Iyy*psi_dot_t*cos(theta_t)*sin(phi_t)^2))/(Iyy*Izz*(sin(theta_t)^2 - 1)), (psi_dot_t*sin(2*phi_t)*(Iyy - Izz)*(Ixx^2*cos(2*theta_t) - Ixx^2 + Ixx*Iyy + Ixx*Izz + Iyy*Izz - Ixx*Iyy*cos(2*theta_t) - Ixx*Izz*cos(2*theta_t) + Iyy*Izz*cos(2*theta_t)))/(4*Ixx*Iyy*Izz),                                                          0,                                                  0;
0, 0, 0, 0, 0, 0, 0, 0, 0, 0, 0, -(Izz^2*theta_dot_t*sin(2*phi_t) - Izz^2*psi_dot_t*cos(theta_t) - Iyy^2*theta_dot_t*sin(2*phi_t) - Iyy^2*psi_dot_t*cos(theta_t) + Ixx*Iyy*psi_dot_t*cos(theta_t) + Ixx*Izz*psi_dot_t*cos(theta_t) + 2*Iyy*Izz*psi_dot_t*cos(theta_t) + Iyy^2*psi_dot_t*cos(2*phi_t)*cos(theta_t) - Izz^2*psi_dot_t*cos(2*phi_t)*cos(theta_t) + Ixx*Iyy*theta_dot_t*sin(2*phi_t) - Ixx*Izz*theta_dot_t*sin(2*phi_t) - Ixx*Iyy*psi_dot_t*cos(2*phi_t)*cos(theta_t) + Ixx*Izz*psi_dot_t*cos(2*phi_t)*cos(theta_t))/(2*Iyy*Izz),                                                                                                                                                                                                                                                                                                                                                                                                                                                                                                                                                                                                                                        -(psi_dot_t*cos(phi_t)*sin(phi_t)*sin(theta_t)*(Iyy - Izz)*(Iyy - Ixx + Izz))/(Iyy*Izz),                           (psi_dot_t*sin(2*theta_t)*(Iyy^2*cos(2*phi_t) - Izz^2*cos(2*phi_t) - Iyy^2 - Izz^2 + Ixx*Iyy + Ixx*Izz - Ixx*Iyy*cos(2*phi_t) + Ixx*Izz*cos(2*phi_t)))/(4*Iyy*Izz),                                                          0,                                                  0;
0, 0, 0, 0, 0, 0, 0, 0, 0, 0, 0,                                            (Ixx*Iyy*theta_dot_t - Izz^2*theta_dot_t - Iyy^2*theta_dot_t + Ixx*Izz*theta_dot_t + 2*Iyy*Izz*theta_dot_t - Iyy^2*theta_dot_t*cos(2*phi_t) + Izz^2*theta_dot_t*cos(2*phi_t) - Iyy^2*psi_dot_t*sin(2*phi_t)*cos(theta_t) + Izz^2*psi_dot_t*sin(2*phi_t)*cos(theta_t) + Ixx*Iyy*theta_dot_t*cos(2*phi_t) - Ixx*Izz*theta_dot_t*cos(2*phi_t) + Ixx*Iyy*psi_dot_t*sin(2*phi_t)*cos(theta_t) - Ixx*Izz*psi_dot_t*sin(2*phi_t)*cos(theta_t))/(2*Iyy*Izz*cos(theta_t)),                                                                                                                                                                                                                                                                                                                                                                                                                                                                                                                                                                                                                  (psi_dot_t*sin(theta_t)*(Iyy - Iyy*sin(phi_t)^2 + Izz*sin(phi_t)^2)*(Iyy - Ixx + Izz))/(Iyy*Izz*cos(theta_t)),                                                                                                       (psi_dot_t*cos(phi_t)*sin(phi_t)*sin(theta_t)*(Iyy - Izz)*(Iyy - Ixx + Izz))/(Iyy*Izz),                                                          0,                                                  0;
0, 0, 0, 0, 0, 0, 0, 0, 0, 0, 0,                                                                                                                                                                                                                                                                                                                                                                                                                                                                                                           0,                                                                                                                                                                                                                                                                                                                                                                                                                                                                                                                                                                                                                                                                                                                              0,                                                                                                                                                                                            0,                     (2*beta_dot_t*sin(beta_t))/cos(beta_t),                                                  0;
0, 0, 0, 0, 0, 0, 0, 0, 0, 0, 0,                                                                                                                                                                                                                                                                                                                                                                                                                                                                                                           0,                                                                                                                                                                                                                                                                                                                                                                                                                                                                                                                                                                                                                                                                                                                              0,                                                                                                                                                                                            0,                             -(alpha_dot_t*sin(2*beta_t))/2,                                                  0];
